simulink model "SSR_naponski_v2"  (R2023b)
settings: Solver=VariableStepAuto  StartTime=0.0  StopTime=10  RelTol=1e-3
undefined symbols (not defined in the file or in its folder): CCM_tf_d_den, CCM_tf_d_num, CCM_tf_i1_den, CCM_tf_i1_num, D0_ccm, D0_dcm, D1, D2, DCM_tf_d_den, DCM_tf_d_num, DCM_tf_i1_den, DCM_tf_i1_num, I10_ccm, I10_dcm, IL0_ccm, IL0_dcm, L, step_time, T, Ubat0_ccm, Ubat0_dcm, Upv0
libraries: simulink_extras x10, dspstat3 x2
settings Model: Creator=teo  LastModifiedBy=teo

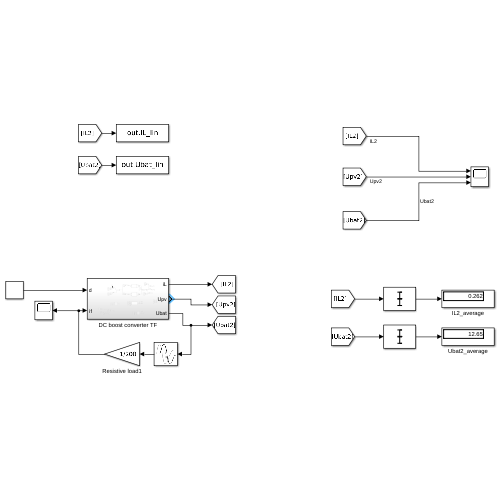
[thumbnail: Simulink's stored preview of the top-level diagram]
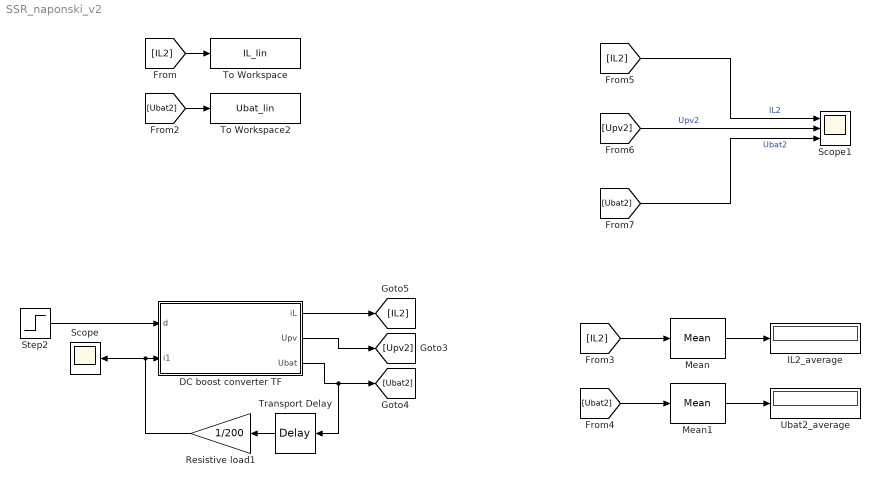
== system SSR_naponski_v2 ==
  DC boost converter TF : Subsystem
  IL2_average : Display
  Mean : dspstat3/Mean  run=off  InputProcessing=Columns as channels (frame based)  reset_popup=None  directionMode=Entire input  dimension=1  roiEnable=off  roiType=Rectangles  roiPortion=Entire ROI  roiOutput=Individual statistics for each ROI  roiFlag=off  roundingMode=Floor  overflowMode=off  outputDataTypeStr=Inherit: Same as accumulator  outputMin=[]  outputMax=[]  outputLastDataTypeStr=Inherit: Same as accumulator
  Mean1 : dspstat3/Mean  run=off  InputProcessing=Columns as channels (frame based)  reset_popup=None  directionMode=Entire input  dimension=1  roiEnable=off  roiType=Rectangles  roiPortion=Entire ROI  roiOutput=Individual statistics for each ROI  roiFlag=off  roundingMode=Floor  overflowMode=off  outputDataTypeStr=Inherit: Same as accumulator  outputMin=[]  outputMax=[]  outputLastDataTypeStr=Inherit: Same as accumulator
  Resistive load1 : Gain  Gain=1/200
  Scope : Scope
  Scope1 : Scope  NumInputPorts=3
  Step2 : Step  Time=step_time  Before=D1  After=D2  SampleTime=0
  To Workspace : ToWorkspace  VariableName=IL_lin  SaveFormat=Timeseries  SampleTime=-1
  To Workspace2 : ToWorkspace  VariableName=Ubat_lin  SaveFormat=Timeseries  SampleTime=-1
  Transport Delay : TransportDelay  DelayTime=0.00001
  Ubat2_average : Display
  wires:
  DC boost converter TF/1(iL) -> [IL2]
  DC boost converter TF/3(Ubat) -> Transport Delay/1, [Ubat2]
  DC boost converter TF/2(Upv) -> [Upv2]
  Resistive load1/1 -> Scope/1, DC boost converter TF/2(i1)
  Step2/1 -> DC boost converter TF/1(d)
  [Upv2] -> Scope1/2  "Upv2"
  [IL2] -> Scope1/1  "IL2"
  [Ubat2] -> Scope1/3  "Ubat2"
  Mean/1 -> IL2_average/1
  [IL2] -> Mean/1
  Mean1/1 -> Ubat2_average/1
  [Ubat2] -> Mean1/1
  [IL2] -> To Workspace/1
  [Ubat2] -> To Workspace2/1
  Transport Delay/1 -> Resistive load1/1

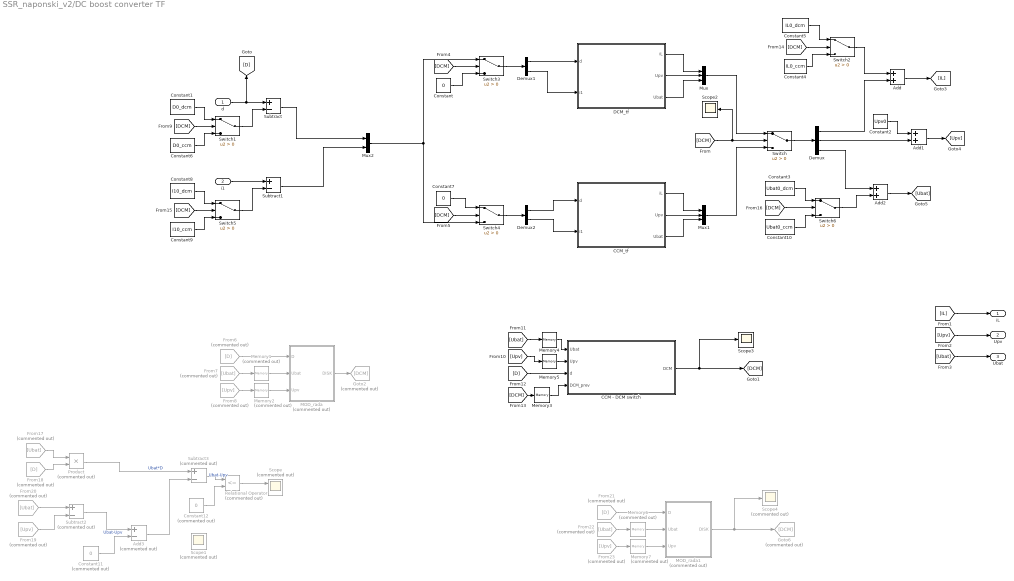
== system SSR_naponski_v2/DC boost converter TF ==
  d : Inport
  i1 : Inport  Port=2
  Add : Sum
  Add1 : Sum
  Add2 : Sum
  Add3 : Sum  Commented=on  Inputs=+-
  CCM - DCM switch : Subsystem
  CCM_tf : Subsystem
  Constant : Constant  Value=0
  Constant1 : Constant  Value=D0_dcm
  Constant10 : Constant  Value=Ubat0_ccm
  Constant11 : Constant  Commented=on  Value=0
  Constant12 : Constant  Commented=on  Value=0
  Constant2 : Constant  Value=Upv0
  Constant3 : Constant  Value=Ubat0_dcm
  Constant4 : Constant  Value=IL0_ccm
  Constant5 : Constant  Value=IL0_dcm
  Constant6 : Constant  Value=D0_ccm
  Constant7 : Constant  Value=0
  Constant8 : Constant  Value=I10_dcm
  Constant9 : Constant  Value=I10_ccm
  DCM_tf : Subsystem
  Demux : Demux  Outputs=3
  Demux1 : Demux  Outputs=2
  Demux2 : Demux  Outputs=2
  From{7,17,20,22} (4 alike) : From  Commented=on  GotoTag=Ubat
  From18 : From  Commented=on  GotoTag=D
  From19 : From  Commented=on  GotoTag=Upv
  From21 : From  Commented=on  GotoTag=D
  From23 : From  Commented=on  GotoTag=Upv
  From6 : From  Commented=on  GotoTag=D
  From8 : From  Commented=on  GotoTag=Upv
  Goto2 : Goto  Commented=on  GotoTag=DCM
  Goto6 : Goto  Commented=on  GotoTag=DCM
  MOD_rada : Subsystem  Commented=on
  MOD_rada1 : Subsystem  Commented=on
  Memory{1..2,6..7} (4 alike) : Memory  Commented=on
  Memory3 : Memory
  Memory4 : Memory
  Memory5 : Memory
  Mux : Mux  Inputs=3
  Mux1 : Mux  Inputs=3
  Mux2 : Mux  Inputs=2
  Product : Product  Commented=on
  Relational Operator : RelationalOperator  Commented=on  Operator=<=  OutDataTypeStr=boolean  RndMeth=Simplest  InputSameDT=off
  Scope : Scope  Commented=on  NumInputPorts=2
  Scope1 : Scope  Commented=on
  Scope2 : Scope
  Scope3 : Scope
  Scope4 : Scope  Commented=on
  Subtract : Sum  Inputs=+-
  Subtract1 : Sum  Inputs=+-
  Subtract2 : Sum  Commented=on  Inputs=+-
  Subtract3 : Sum  Commented=on  Inputs=+-
  Switch{,1..6} (7 alike) : Switch  Criteria=u2 > Threshold  SaturateOnIntegerOverflow=off  InputSameDT=off
  iL : Outport
  Upv : Outport  Port=2
  Ubat : Outport  Port=3
  wires:
  Add1/1 -> [Upv]
  Add2/1 -> [Ubat]
  Add/1 -> [IL]
  [D] -> CCM - DCM switch/3(d)
  DCM_tf/2(Upv) -> Mux/2
  DCM_tf/1(iL) -> Mux/1
  DCM_tf/3(Ubat) -> Mux/3
  CCM_tf/1(iL) -> Mux1/1
  CCM_tf/2(Upv) -> Mux1/2
  CCM_tf/3(Ubat) -> Mux1/3
  Mux1/1 -> Switch/3
  Mux/1 -> Switch/1
  [DCM] -> Switch/2, Scope2/1
  Switch/1 -> Demux/1
  Constant5/1 -> Switch2/1
  Constant4/1 -> Switch2/3
  [DCM] -> Switch2/2
  Switch2/1 -> Add/1
  Demux/1 -> Add/2
  Demux/2 -> Add1/2
  Constant2/1 -> Add1/1
  Demux/3 -> Add2/1
  [IL] -> iL/1
  [Upv] -> Upv/1
  [Ubat] -> Ubat/1
  Constant6/1 -> Switch1/3
  Constant1/1 -> Switch1/1
  [DCM] -> Switch1/2
  Switch3/1 -> Demux1/1
  Demux1/1 -> DCM_tf/1(d)
  Demux1/2 -> DCM_tf/2(i1)
  Demux2/1 -> CCM_tf/1(d)
  Demux2/2 -> CCM_tf/2(i1)
  Switch4/1 -> Demux2/1
  Mux2/1 -> Switch4/3, Switch3/1
  Constant/1 -> Switch3/3
  Constant7/1 -> Switch4/1
  [DCM] -> Switch3/2
  [DCM] -> Switch4/2
  CCM - DCM switch/1(DCM) -> Scope3/1, [DCM]
  MOD_rada/1(DISK) -> Goto2/1
  From6/1 -> MOD_rada/1(D)
  Memory1/1 -> MOD_rada/2(Ubat)
  From7/1 -> Memory1/1
  Memory2/1 -> MOD_rada/3(Upv)
  From8/1 -> Memory2/1
  [Ubat] -> Memory4/1
  [Upv] -> Memory5/1
  Memory5/1 -> CCM - DCM switch/2(Upv)
  Memory4/1 -> CCM - DCM switch/1(Ubat)
  d/1 -> [D], Subtract/1
  Switch1/1 -> Subtract/2
  [DCM] -> Switch5/2
  Constant8/1 -> Switch5/1
  Constant9/1 -> Switch5/3
  Switch5/1 -> Subtract1/2
  Subtract1/1 -> Mux2/2
  i1/1 -> Subtract1/1
  [DCM] -> Memory3/1
  Memory3/1 -> CCM - DCM switch/4(DCM_prev)
  Switch6/1 -> Add2/2
  Constant3/1 -> Switch6/1
  Constant10/1 -> Switch6/3
  [DCM] -> Switch6/2
  Subtract/1 -> Mux2/1
  From17/1 -> Product/1
  From18/1 -> Product/2
  From20/1 -> Subtract2/1
  From19/1 -> Subtract2/2
  Subtract2/1 -> Add3/1  "Ubat-Upv"
  Product/1 -> Subtract3/1  "Ubat*D"
  Constant11/1 -> Add3/2
  Add3/1 -> Subtract3/2
  Subtract3/1 -> Relational Operator/1  "Ubat-Upv"
  Constant12/1 -> Relational Operator/2
  Relational Operator/1 -> Scope/1
  Memory7/1 -> MOD_rada1/3(Upv)
  From21/1 -> MOD_rada1/1(D)
  Memory6/1 -> MOD_rada1/2(Ubat)
  From22/1 -> Memory6/1
  From23/1 -> Memory7/1
  MOD_rada1/1(DISK) -> Scope4/1, Goto6/1

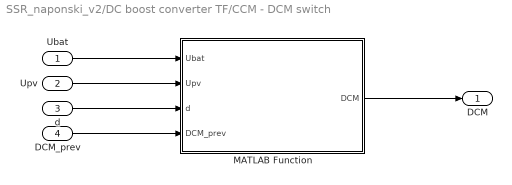
== system SSR_naponski_v2/DC boost converter TF/CCM - DCM switch ==
  Ubat : Inport
  Upv : Inport  Port=2
  d : Inport  Port=3
  DCM_prev : Inport  Port=4
  MATLAB Function : MATLAB Function  TreatAsAtomicUnit=on
  DCM : Outport
  wires:
  MATLAB Function/1(DCM) -> DCM/1
  Ubat/1 -> MATLAB Function/1(Ubat)
  Upv/1 -> MATLAB Function/2(Upv)
  d/1 -> MATLAB Function/3(d)
  DCM_prev/1 -> MATLAB Function/4(DCM_prev)

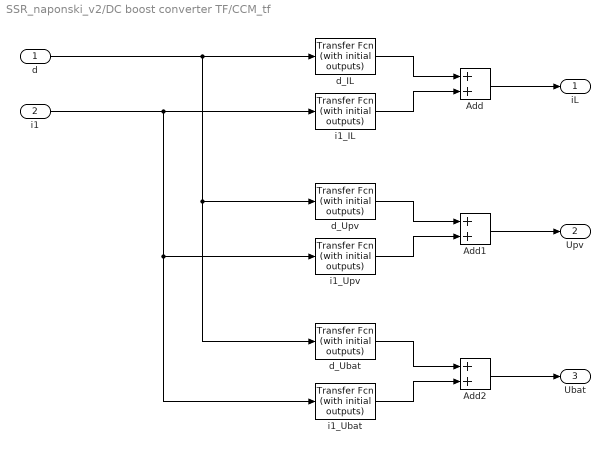
== system SSR_naponski_v2/DC boost converter TF/CCM_tf ==
  d : Inport
  i1 : Inport  Port=2
  Add : Sum
  Add1 : Sum
  Add2 : Sum
  d_IL : simulink_extras/Additional Linear/Transfer Fcn (with initial outputs)  N=CCM_tf_d_num(1, :)  D=CCM_tf_d_den(:)  Y0=0  U0=0
  d_Ubat : simulink_extras/Additional Linear/Transfer Fcn (with initial outputs)  N=CCM_tf_d_num(3, :)  D=CCM_tf_d_den(:)  Y0=0  U0=0
  d_Upv : simulink_extras/Additional Linear/Transfer Fcn (with initial outputs)  N=CCM_tf_d_num(2, :)  D=CCM_tf_d_den(:)  Y0=0  U0=0
  i1_IL : simulink_extras/Additional Linear/Transfer Fcn (with initial outputs)  N=CCM_tf_i1_num(1, :)  D=CCM_tf_i1_den(:)  Y0=0  U0=0
  i1_Ubat : simulink_extras/Additional Linear/Transfer Fcn (with initial outputs)  N=CCM_tf_i1_num(3, :)  D=CCM_tf_i1_den(:)  Y0=0  U0=0
  i1_Upv : simulink_extras/Additional Linear/Transfer Fcn (with initial outputs)  N=CCM_tf_i1_num(2, :)  D=CCM_tf_i1_den(:)  Y0=0  U0=0
  iL : Outport
  Upv : Outport  Port=2
  Ubat : Outport  Port=3
  wires:
  d/1 -> d_Ubat/1, d_Upv/1, d_IL/1
  i1/1 -> i1_Ubat/1, i1_Upv/1, i1_IL/1
  d_IL/1 -> Add/1
  i1_IL/1 -> Add/2
  Add/1 -> iL/1
  d_Upv/1 -> Add1/1
  i1_Upv/1 -> Add1/2
  Add1/1 -> Upv/1
  d_Ubat/1 -> Add2/1
  i1_Ubat/1 -> Add2/2
  Add2/1 -> Ubat/1

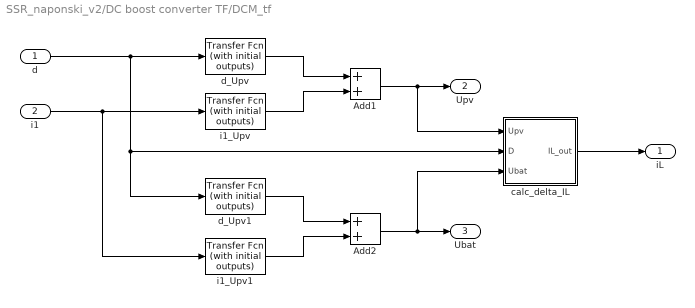
== system SSR_naponski_v2/DC boost converter TF/DCM_tf ==
  d : Inport
  i1 : Inport  Port=2
  Add1 : Sum
  Add2 : Sum
  calc_delta_IL : Subsystem
  d_Upv : simulink_extras/Additional Linear/Transfer Fcn (with initial outputs)  N=DCM_tf_d_num(1, :)  D=DCM_tf_d_den(:)  Y0=0  U0=0
  d_Upv1 : simulink_extras/Additional Linear/Transfer Fcn (with initial outputs)  N=DCM_tf_d_num(2, :)  D=DCM_tf_d_den(:)  Y0=0  U0=0
  i1_Upv : simulink_extras/Additional Linear/Transfer Fcn (with initial outputs)  N=DCM_tf_i1_num(1, :)  D=DCM_tf_i1_den(:)  Y0=0  U0=0
  i1_Upv1 : simulink_extras/Additional Linear/Transfer Fcn (with initial outputs)  N=DCM_tf_i1_num(2, :)  D=DCM_tf_i1_den(:)  Y0=0  U0=0
  iL : Outport
  Upv : Outport  Port=2
  Ubat : Outport  Port=3
  wires:
  d_Upv/1 -> Add1/1
  i1_Upv/1 -> Add1/2
  Add1/1 -> calc_delta_IL/1(Upv), Upv/1
  d_Upv1/1 -> Add2/1
  i1_Upv1/1 -> Add2/2
  Add2/1 -> calc_delta_IL/3(Ubat), Ubat/1
  i1/1 -> i1_Upv1/1, i1_Upv/1
  d/1 -> d_Upv1/1, calc_delta_IL/2(D), d_Upv/1
  calc_delta_IL/1(IL_out) -> iL/1

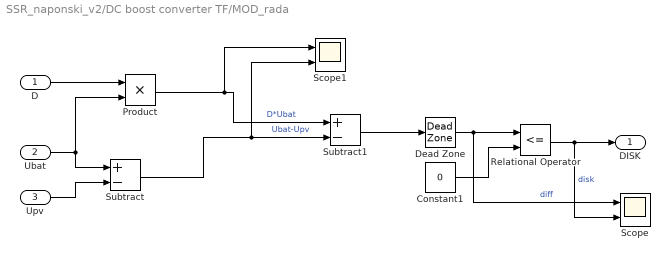
== system SSR_naponski_v2/DC boost converter TF/MOD_rada ==
  D : Inport
  Ubat : Inport  Port=2
  Upv : Inport  Port=3
  Constant1 : Constant  Value=0
  Dead Zone : DeadZone  UpperValue=0
  Product : Product
  Relational Operator : RelationalOperator  Operator=<=  OutDataTypeStr=boolean  RndMeth=Simplest  InputSameDT=off
  Scope : Scope  NumInputPorts=2
  Scope1 : Scope  NumInputPorts=2
  Subtract : Sum  Inputs=+-
  Subtract1 : Sum  Inputs=+-
  DISK : Outport
  wires:
  Ubat/1 -> Product/2, Subtract/1
  Upv/1 -> Subtract/2
  Product/1 -> Scope1/1, Subtract1/1  "D*Ubat"
  D/1 -> Product/1
  Subtract/1 -> Scope1/2, Subtract1/2  "Ubat-Upv"
  Subtract1/1 -> Dead Zone/1
  Dead Zone/1 -> Scope/1, Relational Operator/1  "diff"
  Relational Operator/1 -> Scope/2, DISK/1  "disk"
  Constant1/1 -> Relational Operator/2

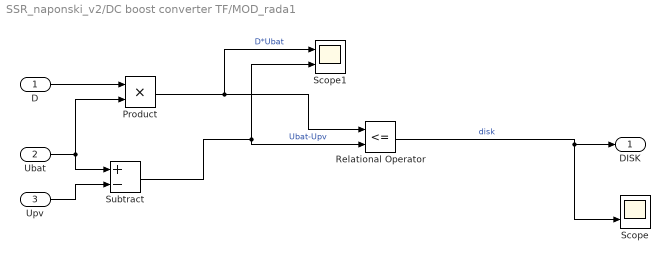
== system SSR_naponski_v2/DC boost converter TF/MOD_rada1 ==
  D : Inport
  Ubat : Inport  Port=2
  Upv : Inport  Port=3
  Product : Product
  Relational Operator : RelationalOperator  Operator=<=  OutDataTypeStr=boolean  RndMeth=Simplest  InputSameDT=off
  Scope : Scope  NumInputPorts=2
  Scope1 : Scope  NumInputPorts=2
  Subtract : Sum  Inputs=+-
  DISK : Outport
  wires:
  Ubat/1 -> Product/2, Subtract/1
  Upv/1 -> Subtract/2
  Product/1 -> Relational Operator/1, Scope1/1  "D*Ubat"
  D/1 -> Product/1
  Subtract/1 -> Relational Operator/2, Scope1/2  "Ubat-Upv"
  Relational Operator/1 -> Scope/2, DISK/1  "disk"

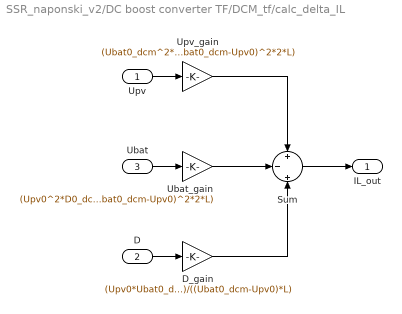
== system SSR_naponski_v2/DC boost converter TF/DCM_tf/calc_delta_IL ==
  Upv : Inport
  D : Inport  Port=2
  Ubat : Inport  Port=3
  D_gain : Gain  Gain=(Upv0*Ubat0_dcm*D0_dcm*T)/((Ubat0_dcm-Upv0)*L)
  Sum : Sum  Inputs=+|-|+
  Ubat_gain : Gain  Gain=(Upv0^2*D0_dcm^2*T)/((Ubat0_dcm-Upv0)^2*2*L)
  Upv_gain : Gain  Gain=(Ubat0_dcm^2*D0_dcm^2*T)/((Ubat0_dcm-Upv0)^2*2*L)
  IL_out : Outport
  wires:
  D/1 -> D_gain/1
  Upv/1 -> Upv_gain/1
  Ubat/1 -> Ubat_gain/1
  Ubat_gain/1 -> Sum/2
  Upv_gain/1 -> Sum/1
  D_gain/1 -> Sum/3
  Sum/1 -> IL_out/1

== matlab function SSR_naponski_v2/DC boost converter TF/CCM - DCM switch/MATLAB Function ==
  data: Ubat input; DCM output; Upv input; d input; DCM_prev input boolean
function DCM = fcn(Ubat, Upv, d, DCM_prev)
        
% Define sensitivity:
err = 1;

if DCM_prev % if in DCM
    if (d * Ubat >= Ubat - Upv + err)
        DCM = false;
    else
        DCM = DCM_prev;
    end
else % if in CCM
    if (d * Ubat <= Ubat - Upv - err)
        DCM = true;
    else
        DCM = DCM_prev;
    end
end
